simulink model "TriggerEdge4_2018a"  (R2018a)
settings: Solver=VariableStepAuto  StartTime=0.0  StopTime=2  RelTol=1e-3
settings Model: Creator=BEAR  LastModifiedBy=bzhan

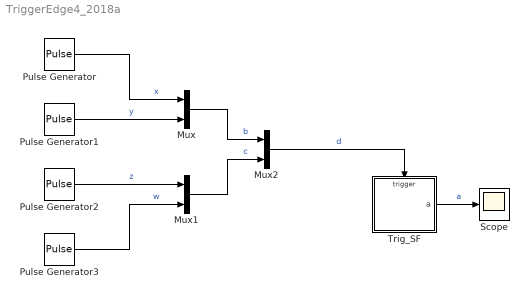
== system TriggerEdge4_2018a ==
  Mux : Mux  Inputs=2
  Mux1 : Mux  Inputs=2
  Mux2 : Mux  Inputs=2
  Pulse Generator : DiscretePulseGenerator  PulseType=Time based  Period=1  PulseWidth=10  PhaseDelay=0.1
  Pulse Generator1 : DiscretePulseGenerator  PulseType=Time based  Period=1  PulseWidth=10  PhaseDelay=0.8
  Pulse Generator2 : DiscretePulseGenerator  PulseType=Time based  Period=1  PulseWidth=10  PhaseDelay=0.3
  Pulse Generator3 : DiscretePulseGenerator  PulseType=Time based  Period=1  PulseWidth=10  PhaseDelay=0.5
  Scope : Scope
  Trig_SF : Stateflow chart  TreatAsAtomicUnit=on
  wires:
  Pulse Generator/1 -> Mux/1  "x"
  Pulse Generator1/1 -> Mux/2  "y"
  Pulse Generator2/1 -> Mux1/1  "z"
  Pulse Generator3/1 -> Mux1/2  "w"
  Mux/1 -> Mux2/1  "b"
  Mux1/1 -> Mux2/2  "c"
  Mux2/1 -> Trig_SF/Trigger  "d"
  Trig_SF/1(a) -> Scope/1  "a"

== stateflow chart TriggerEdge4_2018a/Trig_SF ==
  settings: executeAtInitialization=1
  state A
  state B
    state B1
    state B2
    (default) -> B1
    B1 -> B2 : event2{a = 2;}
    B2 -> B1 : event3{a = 3;}
  (default) -> A
  A -> B : event{a = 0;}
  B -> A : event1{a = 1;}
  data: a output =-1
  events: event input RISING_EDGE_EVENT; event1 input RISING_EDGE_EVENT; event2 input RISING_EDGE_EVENT; event3 input RISING_EDGE_EVENT
